simulink model "power_dcdrive_disc"  (Simulink 7.8)
settings: Solver=FixedStepDiscrete  SolverMode=SingleTasking  StartTime=0.0  StopTime=2  FixedStep=Ts  RelTol=1e-3  AbsTol=1e-3
PreLoadFcn:
  | assignin('base','Ts',[10e-6])
undefined symbols (not defined in the file): Ts
libraries: powerlib x12, powerlib_extras x1
Description:
  | The 'PreLoadFcn' of power_dcdrive_disc.mdl
  | 
  | 
  | automatically sets 'Ts' to 10e-6 in your Workspace.
  | 
  | 
  | Copyright 2008-2011 The MathWorks, Inc.
settings Model: Creator=MathWorks  LastModifiedBy=batserve  ExtModeTrigMode=oneshot  ExtModeArmWhenConnect=off  ExtModeAutoUpdateStatusClock=off
settings DataIOCC: LimitDataPoints=off  SaveFinalState=on  SaveFormat=StructureWithTime  SaveOutput=off  SaveTime=off  SignalLoggingName=sigsOut
settings OptimizationCC: BlockReduction=off  BooleanDataType=off  InlineInvariantSignals=on  InitFltsAndDblsToZero=on
settings DebuggingCC: SaveWithParameterizedLinksMsg=none  CheckExecutionContextPreStartOutputMsg=on  CheckExecutionContextRuntimeOutputMsg=on  SignalResolutionControl=TryResolveAllWithWarning  SolverPrmCheckMsg=none  MultiTaskDSMMsg=warning  MultiTaskCondExecSysMsg=none  FcnCallInpInsideContextMsg=Use local settings  UnconnectedInputMsg=none  UnconnectedOutputMsg=none  StrictBusMsg=None
settings HardwareCC: TargetUnknown=on
settings RTWCC: IncludeERTFirstTime=on
settings GRTTargetCC: TargetFcnLib=ansi_tfl_tmw.mat

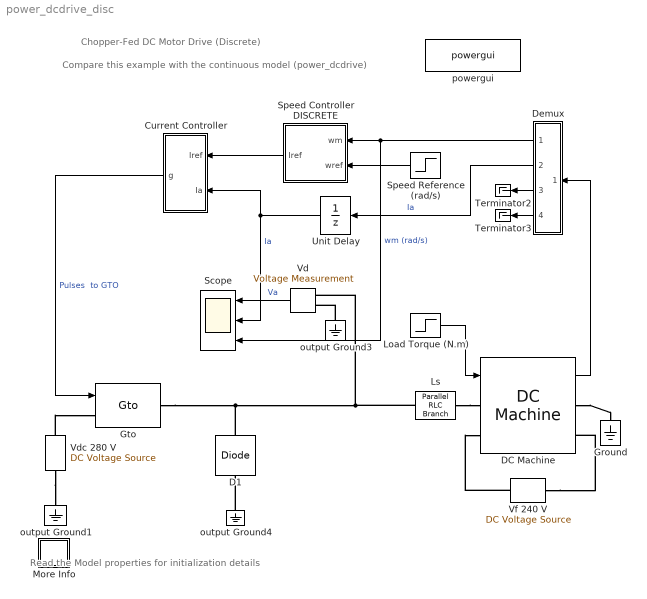
== system power_dcdrive_disc ==
  note: Chopper-Fed DC Motor Drive (Discrete)
  note: Compare this example with the continuous model (power_dcdrive)
  note: Read the Model properties
      | for initialization details
  Current Controller : Subsystem  mask{h=2}
      mask prompts: h "Hysteresis band (A)"
      mask help: Hysteresis Current Controller
      mask Display: plot(0,0,100,100,[45,45],[35,65],[55,55],[35,65],[45,65],[65,65],[35,55],[35,35])
  D1 : powerlib/Power Electronics/Diode  Ron=0.05  Lon=0  Vf=0.7  IC=0  UseSnubber=off  Rs=Inf  Cs=0.1e-6  Measurements=off
  DC Machine : powerlib/Machines/DC Machine  PresetModel=No  MechanicalLoad=Torque TL  FieldType=Wound  ShowDetailedParameters=on  RLa="[0.5  0.01]"  RLf="[ 240  0]"  Laf=1.23  MachineConstant=Torque constant (N.m/A)  Ke=1.8  Kt=1.8  J=0.05  Bm=0.02  Tf=0  w0=0  Ifinit=1  TsPowergui=0  TsBlock=-1
      settings: AttributesFormatString=\n
  Demux : Subsystem
  Ground : powerlib/Elements/Ground  LConnTagsString=a
  Gto : powerlib/Power Electronics/Gto  Ron=0.05  Lon=0  Vf=1  Tf=1e-6  Tt=1e-6  IC=0  Rs=1e4  Cs=inf  Measurements=off
      settings: AttributesFormatString=\n
  "Load Torque (N.m) " : Step  Time=1.5  Before=5  After=25  SampleTime=0
  Ls : powerlib/Elements/Parallel RLC Branch  LConnTagsString=a  RConnTagsString=__new0  BranchType=L  Resistance=1.0  Inductance=10e-03  SetiL0=off  InitialCurrent=0  Capacitance=1.0  Setx0=off  InitialVoltage=0  Measurements=None
  More Info : Subsystem
      settings: OpenFcn=showdemo(bdroot(gcb))
      mask Display: disp('?')
  Scope : Scope  NumInputPorts=3
      settings: TickLabels=on  TimeRange=2  YMin=-100~0~-50  YMax=400~40~200  SaveName=var
  Speed Controller DISCRETE : Subsystem  mask(PI controller){Kp=1.6, Ki=16, Ilim=30, Ts=Ts}
      mask prompts: Kp "Proportional gain (Kp)"; Ki "Integral gain (Ki)"; Ilim "Current limit (A)"; Ts "Sample time (s) :"
      mask help: Proportional-Integral Speed Controller
      mask Display: plot(0,0,100,100,[35,35,65],[70,30,30],[35,65],[45,60])
  Speed Reference (rad/s) : Step  Time=0.8  Before=120  After=160  SampleTime=0
  Terminator2 : Terminator
  Terminator3 : Terminator
  Unit Delay : UnitDelay  SampleTime=Ts
  Vd : powerlib/Measurements/Voltage Measurement  Tag=PoWeRsYsTeMmEaSuReMeNt  PhasorSimulation=off  OutputType=Magnitude  PSBequivalent=0
  "Vdc 280 V " : powerlib/Electrical Sources/DC Voltage Source  Description=source block  Amplitude=280  Measurements=None
      settings: AttributesFormatString=\n
  Vf 240 V : powerlib/Electrical Sources/DC Voltage Source  Description=source block  Amplitude=240  Measurements=None
      settings: AttributesFormatString=\n
  output Ground1 : powerlib/Elements/Ground  LConnTagsString=a
  output Ground3 : powerlib/Elements/Ground  LConnTagsString=a
  output Ground4 : powerlib/Elements/Ground  LConnTagsString=a
  powergui : powerlib/powergui  Priority=2  SimulationMode=Discrete  SolverType=Tustin  SampleTime=10e-6  frequency=60  SPID=off  DisableSnubberDevices=off  DisableRonSwitches=off  DisableVfSwitches=off  SwTol=0  Interpol=off  DisplayEquations=off  FunctionMessages=off  frequencyindice=1  Pbase=100e6  ErrMax=1e-4  Iterations=50  UnitsV=kV  UnitsW=MW  echomessages=off  HookPort=off  EnableUseOfTLC=off  x0status=blocks  RestoreLinks=warning  ResistiveCurrentMeasurement=off  Frange=[0:2:500]  Ylog=off  Xlog=on  ShowGrid=off  save=off  variable=ZData  ZoomFFT=on  StartTime=0.0  cycles=1  DisplayStyle=off  fundamental=60  FreqAxis=off  MaxFrequency=1000  frequencyindicesteady=1  RmsSteady=1  display=off  Ts=0  methode=off
  wires:
  Speed Controller DISCRETE/1(Iref) -> Current Controller/1(Iref)
  Demux/1(wm) -> Speed Controller DISCRETE/1(wm), Scope/3  "wm (rad/s)"
  Demux/2(Ia) -> Unit Delay/1  "Ia"
  Demux/4(Te) -> Terminator3/1
  Demux/3(If) -> Terminator2/1
  Current Controller/1(g) -> Gto/1  "Pulses  to GTO"
  Speed Reference (rad/s)/1 -> Speed Controller DISCRETE/2(wref)
  Vd/1 -> Scope/1  "Va"
  "Load Torque (N.m) "/1 -> DC Machine/1
  Unit Delay/1 -> Current Controller/2(Ia), Scope/2  "Ia"
  DC Machine/1 -> Demux/1(m)
  connections:
  "Vdc 280 V "/RConn1 -- Gto/LConn1
  "Vdc 280 V "/LConn1 -- output Ground1/LConn1
  Ls/RConn1 -- DC Machine/LConn1
  DC Machine/RConn1 -- Ground/LConn1
  D1/RConn1 -- Ls/LConn1 -- Vd/LConn1 -- Gto/RConn1
  output Ground3/LConn1 -- Vd/LConn2
  Vf 240 V/LConn1 -- DC Machine/RConn2
  Vf 240 V/RConn1 -- DC Machine/LConn2
  output Ground4/LConn1 -- D1/LConn1

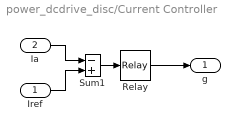
== system power_dcdrive_disc/Current Controller ==
  Iref : Inport
  Ia : Inport  Port=2
  Relay : Relay  OnSwitchValue=h/2  OffSwitchValue=-h/2
  Sum1 : Sum  Inputs=-+  SaturateOnIntegerOverflow=on  InputSameDT=on  OutDataTypeStr=Inherit: Same as first input
  g : Outport  InitialOutput=0
  wires:
  Sum1/1 -> Relay/1
  Relay/1 -> g/1
  Ia/1 -> Sum1/1
  Iref/1 -> Sum1/2

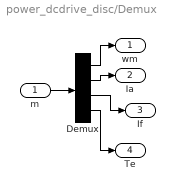
== system power_dcdrive_disc/Demux ==
  m : Inport
  Demux : Demux
  wm : Outport
  Ia : Outport  Port=2
  If : Outport  Port=3
  Te : Outport  Port=4
  wires:
  Demux/1 -> wm/1
  Demux/2 -> Ia/1
  m/1 -> Demux/1
  Demux/3 -> If/1
  Demux/4 -> Te/1

== system power_dcdrive_disc/More Info ==

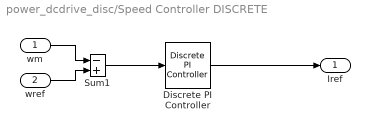
== system power_dcdrive_disc/Speed Controller DISCRETE ==
  wm : Inport
  wref : Inport  Port=2
  Discrete PI Controller : powerlib_extras/Discrete  Control Blocks/Discrete PI Controller  Kp=Kp  Ki=Ki  Par_Limits=[Ilim -Ilim]  Init=0  Ts=Ts
  Sum1 : Sum  Inputs=-+  SaturateOnIntegerOverflow=on  InputSameDT=on  OutDataTypeStr=Inherit: Same as first input
  Iref : Outport  InitialOutput=0
  wires:
  wref/1 -> Sum1/2
  wm/1 -> Sum1/1
  Sum1/1 -> Discrete PI Controller/1
  Discrete PI Controller/1 -> Iref/1
